simulink model "exampleMinRunTime3"  (R2016b)
settings: Solver=ode45  StartTime=0.0  StopTime=30  RelTol=1e-3  EnableMultiTasking=on
libraries: simulink x1
settings Model: Creator=drhf  LastModifiedBy=drhf
settings DataIOCC: LimitDataPoints=on  SaveFormat=Array  SignalLoggingSaveFormat=ModelDataLogs
settings OptimizationCC: ExpressionDepthLimit=2147483647  LifeSpan=inf
settings DebuggingCC: UnderspecifiedInitializationDetection=Classic  MergeDetectMultiDrivingBlocksExec=none  SolverPrmCheckMsg=warning  StateNameClashWarn=warning  SFUnexpectedBacktrackingDiag=warning  SFNoUnconditionalDefaultTransitionDiag=warning  SFExecutionAtInitializationDiag=none
settings HardwareCC: ProdBitPerPointer=32  ProdBitPerSizeT=32  ProdBitPerPtrDiffT=32  ProdLargestAtomicFloat=None  ProdIntDivRoundTo=Undefined  ProdEndianess=Unspecified  ProdWordSize=32  ProdHWDeviceType=32-bit Generic
settings ModelReferenceCC: PropagateSignalLabelsOutOfModel=off
settings GRTTargetCC: TargetLangStandard=C89/C90 (ANSI)  GeneratePreprocessorConditionals=Disable all  CombineOutputUpdateFcns=off  GRTInterface=on
settings ConfigComp: CovMetricSettings=dw  CovHtmlReporting=on  CovSaveCumulativeToWorkspaceVar=on  CovSaveSingleToWorkspaceVar=on  CovExternalEMLEnable=off

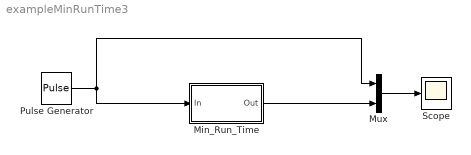
== system exampleMinRunTime3 ==
  Min_Run_Time : Subsystem
  Mux : Mux  Inputs=2
  Pulse Generator : DiscretePulseGenerator  PulseType=Time based  Amplitude=2  Period=10  PulseWidth=5
  Scope : Scope
  wires:
  Pulse Generator/1 -> Mux/1, Min_Run_Time/1(In)
  Mux/1 -> Scope/1
  Min_Run_Time/1(Out) -> Mux/2

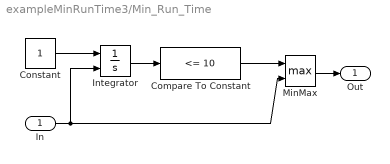
== system exampleMinRunTime3/Min_Run_Time ==
  In : Inport
  Compare To Constant : simulink/Logic and Bit Operations/Compare To Constant  relop=<=  const=10  OutDataTypeStr=uint8
  Constant : Constant
  Integrator : Integrator  ExternalReset=rising
  MinMax : MinMax  Function=max  Inputs=2
  Out : Outport
  wires:
  Constant/1 -> Integrator/1
  Integrator/1 -> Compare To Constant/1
  MinMax/1 -> Out/1
  In/1 -> Integrator/2, MinMax/2
  Compare To Constant/1 -> MinMax/1
